simulink model "gm_parallel_lht"  (R2019b)
settings: Solver=FixedStepDiscrete  StartTime=0.0  StopTime=inf  RelTol=1e-3
undefined symbols (not defined in the file or in its folder): bt, height, width
libraries: hdlsllib x190, simulink x13, hdlmdlgenlib x7, dspsrcs4 x1
(part 17 of 18)

== system gm_parallel_lht/Parallel LHT/Parallel LHT Kernel/Hough Kernel/Hough Kernel Symmetric Look Ahead/Look Ahead Hough/Register Bank_instance42 ==
  Data In : Inport  OutDataTypeStr=fixdt(1, 11, 0)  PortDimensions=1  SampleTime=6.66666666666667e-09
  Write Enable : Inport  Port=2  OutDataTypeStr=boolean  PortDimensions=1  SampleTime=6.66666666666667e-09
  Delay_Switch : Switch  Criteria=u2 ~= 0  Threshold=double(0)  OutDataTypeStr=fixdt(1, 11, 0)  SampleTime=6.66666666666667e-09
  Unit Delay Enabled Synchronous_lowered : Delay  DelayLength=double(1)  InitialCondition=0  SampleTime=6.66666666666667e-09
  Data Out : Outport
  wires:
  Delay_Switch/1 -> Unit Delay Enabled Synchronous_lowered/1
  Write Enable/1 -> Delay_Switch/2
  Data In/1 -> Delay_Switch/1
  Unit Delay Enabled Synchronous_lowered/1 -> Delay_Switch/3, Data Out/1

== system gm_parallel_lht/Parallel LHT/Parallel LHT Kernel/Hough Kernel/Hough Kernel Symmetric Look Ahead/Look Ahead Hough/Register Bank_instance43 ==
  Data In : Inport  OutDataTypeStr=fixdt(1, 11, 0)  PortDimensions=1  SampleTime=6.66666666666667e-09
  Write Enable : Inport  Port=2  OutDataTypeStr=boolean  PortDimensions=1  SampleTime=6.66666666666667e-09
  Delay_Switch : Switch  Criteria=u2 ~= 0  Threshold=double(0)  OutDataTypeStr=fixdt(1, 11, 0)  SampleTime=6.66666666666667e-09
  Unit Delay Enabled Synchronous_lowered : Delay  DelayLength=double(1)  InitialCondition=0  SampleTime=6.66666666666667e-09
  Data Out : Outport
  wires:
  Delay_Switch/1 -> Unit Delay Enabled Synchronous_lowered/1
  Write Enable/1 -> Delay_Switch/2
  Data In/1 -> Delay_Switch/1
  Unit Delay Enabled Synchronous_lowered/1 -> Delay_Switch/3, Data Out/1

== system gm_parallel_lht/Parallel LHT/Parallel LHT Kernel/Hough Kernel/Hough Kernel Symmetric Look Ahead/Look Ahead Hough/Register Bank_instance44 ==
  Data In : Inport  OutDataTypeStr=fixdt(1, 11, 0)  PortDimensions=1  SampleTime=6.66666666666667e-09
  Write Enable : Inport  Port=2  OutDataTypeStr=boolean  PortDimensions=1  SampleTime=6.66666666666667e-09
  Delay_Switch : Switch  Criteria=u2 ~= 0  Threshold=double(0)  OutDataTypeStr=fixdt(1, 11, 0)  SampleTime=6.66666666666667e-09
  Unit Delay Enabled Synchronous_lowered : Delay  DelayLength=double(1)  InitialCondition=0  SampleTime=6.66666666666667e-09
  Data Out : Outport
  wires:
  Delay_Switch/1 -> Unit Delay Enabled Synchronous_lowered/1
  Write Enable/1 -> Delay_Switch/2
  Data In/1 -> Delay_Switch/1
  Unit Delay Enabled Synchronous_lowered/1 -> Delay_Switch/3, Data Out/1

== system gm_parallel_lht/Parallel LHT/Parallel LHT Kernel/Hough Kernel/Hough Kernel Symmetric Look Ahead/Look Ahead Hough/Register Bank_instance45 ==
  Data In : Inport  OutDataTypeStr=fixdt(1, 11, 0)  PortDimensions=1  SampleTime=6.66666666666667e-09
  Write Enable : Inport  Port=2  OutDataTypeStr=boolean  PortDimensions=1  SampleTime=6.66666666666667e-09
  Delay_Switch : Switch  Criteria=u2 ~= 0  Threshold=double(0)  OutDataTypeStr=fixdt(1, 11, 0)  SampleTime=6.66666666666667e-09
  Unit Delay Enabled Synchronous_lowered : Delay  DelayLength=double(1)  InitialCondition=0  SampleTime=6.66666666666667e-09
  Data Out : Outport
  wires:
  Delay_Switch/1 -> Unit Delay Enabled Synchronous_lowered/1
  Write Enable/1 -> Delay_Switch/2
  Data In/1 -> Delay_Switch/1
  Unit Delay Enabled Synchronous_lowered/1 -> Delay_Switch/3, Data Out/1

== system gm_parallel_lht/Parallel LHT/Parallel LHT Kernel/Hough Kernel/Hough Kernel Symmetric Look Ahead/Look Ahead Hough/Register Bank_instance46 ==
  Data In : Inport  OutDataTypeStr=fixdt(1, 11, 0)  PortDimensions=1  SampleTime=6.66666666666667e-09
  Write Enable : Inport  Port=2  OutDataTypeStr=boolean  PortDimensions=1  SampleTime=6.66666666666667e-09
  Delay_Switch : Switch  Criteria=u2 ~= 0  Threshold=double(0)  OutDataTypeStr=fixdt(1, 11, 0)  SampleTime=6.66666666666667e-09
  Unit Delay Enabled Synchronous_lowered : Delay  DelayLength=double(1)  InitialCondition=0  SampleTime=6.66666666666667e-09
  Data Out : Outport
  wires:
  Delay_Switch/1 -> Unit Delay Enabled Synchronous_lowered/1
  Write Enable/1 -> Delay_Switch/2
  Data In/1 -> Delay_Switch/1
  Unit Delay Enabled Synchronous_lowered/1 -> Delay_Switch/3, Data Out/1

== system gm_parallel_lht/Parallel LHT/Parallel LHT Kernel/Hough Kernel/Hough Kernel Symmetric Look Ahead/Look Ahead Hough/Register Bank_instance47 ==
  Data In : Inport  OutDataTypeStr=fixdt(1, 11, 0)  PortDimensions=1  SampleTime=6.66666666666667e-09
  Write Enable : Inport  Port=2  OutDataTypeStr=boolean  PortDimensions=1  SampleTime=6.66666666666667e-09
  Delay_Switch : Switch  Criteria=u2 ~= 0  Threshold=double(0)  OutDataTypeStr=fixdt(1, 11, 0)  SampleTime=6.66666666666667e-09
  Unit Delay Enabled Synchronous_lowered : Delay  DelayLength=double(1)  InitialCondition=0  SampleTime=6.66666666666667e-09
  Data Out : Outport
  wires:
  Delay_Switch/1 -> Unit Delay Enabled Synchronous_lowered/1
  Write Enable/1 -> Delay_Switch/2
  Data In/1 -> Delay_Switch/1
  Unit Delay Enabled Synchronous_lowered/1 -> Delay_Switch/3, Data Out/1

== system gm_parallel_lht/Parallel LHT/Parallel LHT Kernel/Hough Kernel/Hough Kernel Symmetric Look Ahead/Look Ahead Hough/Register Bank_instance48 ==
  Data In : Inport  OutDataTypeStr=fixdt(1, 11, 0)  PortDimensions=1  SampleTime=6.66666666666667e-09
  Write Enable : Inport  Port=2  OutDataTypeStr=boolean  PortDimensions=1  SampleTime=6.66666666666667e-09
  Delay_Switch : Switch  Criteria=u2 ~= 0  Threshold=double(0)  OutDataTypeStr=fixdt(1, 11, 0)  SampleTime=6.66666666666667e-09
  Unit Delay Enabled Synchronous_lowered : Delay  DelayLength=double(1)  InitialCondition=0  SampleTime=6.66666666666667e-09
  Data Out : Outport
  wires:
  Delay_Switch/1 -> Unit Delay Enabled Synchronous_lowered/1
  Write Enable/1 -> Delay_Switch/2
  Data In/1 -> Delay_Switch/1
  Unit Delay Enabled Synchronous_lowered/1 -> Delay_Switch/3, Data Out/1

== system gm_parallel_lht/Parallel LHT/Parallel LHT Kernel/Hough Kernel/Hough Kernel Symmetric Look Ahead/Look Ahead Hough/Register Bank_instance49 ==
  Data In : Inport  OutDataTypeStr=fixdt(1, 11, 0)  PortDimensions=1  SampleTime=6.66666666666667e-09
  Write Enable : Inport  Port=2  OutDataTypeStr=boolean  PortDimensions=1  SampleTime=6.66666666666667e-09
  Delay_Switch : Switch  Criteria=u2 ~= 0  Threshold=double(0)  OutDataTypeStr=fixdt(1, 11, 0)  SampleTime=6.66666666666667e-09
  Unit Delay Enabled Synchronous_lowered : Delay  DelayLength=double(1)  InitialCondition=0  SampleTime=6.66666666666667e-09
  Data Out : Outport
  wires:
  Delay_Switch/1 -> Unit Delay Enabled Synchronous_lowered/1
  Write Enable/1 -> Delay_Switch/2
  Data In/1 -> Delay_Switch/1
  Unit Delay Enabled Synchronous_lowered/1 -> Delay_Switch/3, Data Out/1

== system gm_parallel_lht/Parallel LHT/Parallel LHT Kernel/Hough Kernel/Hough Kernel Symmetric Look Ahead/Look Ahead Hough/Register Bank_instance5 ==
  Data In : Inport  OutDataTypeStr=fixdt(1, 11, 0)  PortDimensions=1  SampleTime=6.66666666666667e-09
  Write Enable : Inport  Port=2  OutDataTypeStr=boolean  PortDimensions=1  SampleTime=6.66666666666667e-09
  Delay_Switch : Switch  Criteria=u2 ~= 0  Threshold=double(0)  OutDataTypeStr=fixdt(1, 11, 0)  SampleTime=6.66666666666667e-09
  Unit Delay Enabled Synchronous_lowered : Delay  DelayLength=double(1)  InitialCondition=0  SampleTime=6.66666666666667e-09
  Data Out : Outport
  wires:
  Delay_Switch/1 -> Unit Delay Enabled Synchronous_lowered/1
  Write Enable/1 -> Delay_Switch/2
  Data In/1 -> Delay_Switch/1
  Unit Delay Enabled Synchronous_lowered/1 -> Delay_Switch/3, Data Out/1

== system gm_parallel_lht/Parallel LHT/Parallel LHT Kernel/Hough Kernel/Hough Kernel Symmetric Look Ahead/Look Ahead Hough/Register Bank_instance50 ==
  Data In : Inport  OutDataTypeStr=fixdt(1, 11, 0)  PortDimensions=1  SampleTime=6.66666666666667e-09
  Write Enable : Inport  Port=2  OutDataTypeStr=boolean  PortDimensions=1  SampleTime=6.66666666666667e-09
  Delay_Switch : Switch  Criteria=u2 ~= 0  Threshold=double(0)  OutDataTypeStr=fixdt(1, 11, 0)  SampleTime=6.66666666666667e-09
  Unit Delay Enabled Synchronous_lowered : Delay  DelayLength=double(1)  InitialCondition=0  SampleTime=6.66666666666667e-09
  Data Out : Outport
  wires:
  Delay_Switch/1 -> Unit Delay Enabled Synchronous_lowered/1
  Write Enable/1 -> Delay_Switch/2
  Data In/1 -> Delay_Switch/1
  Unit Delay Enabled Synchronous_lowered/1 -> Delay_Switch/3, Data Out/1

== system gm_parallel_lht/Parallel LHT/Parallel LHT Kernel/Hough Kernel/Hough Kernel Symmetric Look Ahead/Look Ahead Hough/Register Bank_instance51 ==
  Data In : Inport  OutDataTypeStr=fixdt(1, 11, 0)  PortDimensions=1  SampleTime=6.66666666666667e-09
  Write Enable : Inport  Port=2  OutDataTypeStr=boolean  PortDimensions=1  SampleTime=6.66666666666667e-09
  Delay_Switch : Switch  Criteria=u2 ~= 0  Threshold=double(0)  OutDataTypeStr=fixdt(1, 11, 0)  SampleTime=6.66666666666667e-09
  Unit Delay Enabled Synchronous_lowered : Delay  DelayLength=double(1)  InitialCondition=0  SampleTime=6.66666666666667e-09
  Data Out : Outport
  wires:
  Delay_Switch/1 -> Unit Delay Enabled Synchronous_lowered/1
  Write Enable/1 -> Delay_Switch/2
  Data In/1 -> Delay_Switch/1
  Unit Delay Enabled Synchronous_lowered/1 -> Delay_Switch/3, Data Out/1

== system gm_parallel_lht/Parallel LHT/Parallel LHT Kernel/Hough Kernel/Hough Kernel Symmetric Look Ahead/Look Ahead Hough/Register Bank_instance52 ==
  Data In : Inport  OutDataTypeStr=fixdt(1, 11, 0)  PortDimensions=1  SampleTime=6.66666666666667e-09
  Write Enable : Inport  Port=2  OutDataTypeStr=boolean  PortDimensions=1  SampleTime=6.66666666666667e-09
  Delay_Switch : Switch  Criteria=u2 ~= 0  Threshold=double(0)  OutDataTypeStr=fixdt(1, 11, 0)  SampleTime=6.66666666666667e-09
  Unit Delay Enabled Synchronous_lowered : Delay  DelayLength=double(1)  InitialCondition=0  SampleTime=6.66666666666667e-09
  Data Out : Outport
  wires:
  Delay_Switch/1 -> Unit Delay Enabled Synchronous_lowered/1
  Write Enable/1 -> Delay_Switch/2
  Data In/1 -> Delay_Switch/1
  Unit Delay Enabled Synchronous_lowered/1 -> Delay_Switch/3, Data Out/1

== system gm_parallel_lht/Parallel LHT/Parallel LHT Kernel/Hough Kernel/Hough Kernel Symmetric Look Ahead/Look Ahead Hough/Register Bank_instance53 ==
  Data In : Inport  OutDataTypeStr=fixdt(1, 11, 0)  PortDimensions=1  SampleTime=6.66666666666667e-09
  Write Enable : Inport  Port=2  OutDataTypeStr=boolean  PortDimensions=1  SampleTime=6.66666666666667e-09
  Delay_Switch : Switch  Criteria=u2 ~= 0  Threshold=double(0)  OutDataTypeStr=fixdt(1, 11, 0)  SampleTime=6.66666666666667e-09
  Unit Delay Enabled Synchronous_lowered : Delay  DelayLength=double(1)  InitialCondition=0  SampleTime=6.66666666666667e-09
  Data Out : Outport
  wires:
  Delay_Switch/1 -> Unit Delay Enabled Synchronous_lowered/1
  Write Enable/1 -> Delay_Switch/2
  Data In/1 -> Delay_Switch/1
  Unit Delay Enabled Synchronous_lowered/1 -> Delay_Switch/3, Data Out/1

== system gm_parallel_lht/Parallel LHT/Parallel LHT Kernel/Hough Kernel/Hough Kernel Symmetric Look Ahead/Look Ahead Hough/Register Bank_instance54 ==
  Data In : Inport  OutDataTypeStr=fixdt(1, 11, 0)  PortDimensions=1  SampleTime=6.66666666666667e-09
  Write Enable : Inport  Port=2  OutDataTypeStr=boolean  PortDimensions=1  SampleTime=6.66666666666667e-09
  Delay_Switch : Switch  Criteria=u2 ~= 0  Threshold=double(0)  OutDataTypeStr=fixdt(1, 11, 0)  SampleTime=6.66666666666667e-09
  Unit Delay Enabled Synchronous_lowered : Delay  DelayLength=double(1)  InitialCondition=0  SampleTime=6.66666666666667e-09
  Data Out : Outport
  wires:
  Delay_Switch/1 -> Unit Delay Enabled Synchronous_lowered/1
  Write Enable/1 -> Delay_Switch/2
  Data In/1 -> Delay_Switch/1
  Unit Delay Enabled Synchronous_lowered/1 -> Delay_Switch/3, Data Out/1

== system gm_parallel_lht/Parallel LHT/Parallel LHT Kernel/Hough Kernel/Hough Kernel Symmetric Look Ahead/Look Ahead Hough/Register Bank_instance55 ==
  Data In : Inport  OutDataTypeStr=fixdt(1, 11, 0)  PortDimensions=1  SampleTime=6.66666666666667e-09
  Write Enable : Inport  Port=2  OutDataTypeStr=boolean  PortDimensions=1  SampleTime=6.66666666666667e-09
  Delay_Switch : Switch  Criteria=u2 ~= 0  Threshold=double(0)  OutDataTypeStr=fixdt(1, 11, 0)  SampleTime=6.66666666666667e-09
  Unit Delay Enabled Synchronous_lowered : Delay  DelayLength=double(1)  InitialCondition=0  SampleTime=6.66666666666667e-09
  Data Out : Outport
  wires:
  Delay_Switch/1 -> Unit Delay Enabled Synchronous_lowered/1
  Write Enable/1 -> Delay_Switch/2
  Data In/1 -> Delay_Switch/1
  Unit Delay Enabled Synchronous_lowered/1 -> Delay_Switch/3, Data Out/1

== system gm_parallel_lht/Parallel LHT/Parallel LHT Kernel/Hough Kernel/Hough Kernel Symmetric Look Ahead/Look Ahead Hough/Register Bank_instance56 ==
  Data In : Inport  OutDataTypeStr=fixdt(1, 11, 0)  PortDimensions=1  SampleTime=6.66666666666667e-09
  Write Enable : Inport  Port=2  OutDataTypeStr=boolean  PortDimensions=1  SampleTime=6.66666666666667e-09
  Delay_Switch : Switch  Criteria=u2 ~= 0  Threshold=double(0)  OutDataTypeStr=fixdt(1, 11, 0)  SampleTime=6.66666666666667e-09
  Unit Delay Enabled Synchronous_lowered : Delay  DelayLength=double(1)  InitialCondition=0  SampleTime=6.66666666666667e-09
  Data Out : Outport
  wires:
  Delay_Switch/1 -> Unit Delay Enabled Synchronous_lowered/1
  Write Enable/1 -> Delay_Switch/2
  Data In/1 -> Delay_Switch/1
  Unit Delay Enabled Synchronous_lowered/1 -> Delay_Switch/3, Data Out/1

== system gm_parallel_lht/Parallel LHT/Parallel LHT Kernel/Hough Kernel/Hough Kernel Symmetric Look Ahead/Look Ahead Hough/Register Bank_instance57 ==
  Data In : Inport  OutDataTypeStr=fixdt(1, 11, 0)  PortDimensions=1  SampleTime=6.66666666666667e-09
  Write Enable : Inport  Port=2  OutDataTypeStr=boolean  PortDimensions=1  SampleTime=6.66666666666667e-09
  Delay_Switch : Switch  Criteria=u2 ~= 0  Threshold=double(0)  OutDataTypeStr=fixdt(1, 11, 0)  SampleTime=6.66666666666667e-09
  Unit Delay Enabled Synchronous_lowered : Delay  DelayLength=double(1)  InitialCondition=0  SampleTime=6.66666666666667e-09
  Data Out : Outport
  wires:
  Delay_Switch/1 -> Unit Delay Enabled Synchronous_lowered/1
  Write Enable/1 -> Delay_Switch/2
  Data In/1 -> Delay_Switch/1
  Unit Delay Enabled Synchronous_lowered/1 -> Delay_Switch/3, Data Out/1

== system gm_parallel_lht/Parallel LHT/Parallel LHT Kernel/Hough Kernel/Hough Kernel Symmetric Look Ahead/Look Ahead Hough/Register Bank_instance58 ==
  Data In : Inport  OutDataTypeStr=fixdt(1, 11, 0)  PortDimensions=1  SampleTime=6.66666666666667e-09
  Write Enable : Inport  Port=2  OutDataTypeStr=boolean  PortDimensions=1  SampleTime=6.66666666666667e-09
  Delay_Switch : Switch  Criteria=u2 ~= 0  Threshold=double(0)  OutDataTypeStr=fixdt(1, 11, 0)  SampleTime=6.66666666666667e-09
  Unit Delay Enabled Synchronous_lowered : Delay  DelayLength=double(1)  InitialCondition=0  SampleTime=6.66666666666667e-09
  Data Out : Outport
  wires:
  Delay_Switch/1 -> Unit Delay Enabled Synchronous_lowered/1
  Write Enable/1 -> Delay_Switch/2
  Data In/1 -> Delay_Switch/1
  Unit Delay Enabled Synchronous_lowered/1 -> Delay_Switch/3, Data Out/1

== system gm_parallel_lht/Parallel LHT/Parallel LHT Kernel/Hough Kernel/Hough Kernel Symmetric Look Ahead/Look Ahead Hough/Register Bank_instance59 ==
  Data In : Inport  OutDataTypeStr=fixdt(1, 11, 0)  PortDimensions=1  SampleTime=6.66666666666667e-09
  Write Enable : Inport  Port=2  OutDataTypeStr=boolean  PortDimensions=1  SampleTime=6.66666666666667e-09
  Delay_Switch : Switch  Criteria=u2 ~= 0  Threshold=double(0)  OutDataTypeStr=fixdt(1, 11, 0)  SampleTime=6.66666666666667e-09
  Unit Delay Enabled Synchronous_lowered : Delay  DelayLength=double(1)  InitialCondition=0  SampleTime=6.66666666666667e-09
  Data Out : Outport
  wires:
  Delay_Switch/1 -> Unit Delay Enabled Synchronous_lowered/1
  Write Enable/1 -> Delay_Switch/2
  Data In/1 -> Delay_Switch/1
  Unit Delay Enabled Synchronous_lowered/1 -> Delay_Switch/3, Data Out/1

== system gm_parallel_lht/Parallel LHT/Parallel LHT Kernel/Hough Kernel/Hough Kernel Symmetric Look Ahead/Look Ahead Hough/Register Bank_instance6 ==
  Data In : Inport  OutDataTypeStr=fixdt(1, 11, 0)  PortDimensions=1  SampleTime=6.66666666666667e-09
  Write Enable : Inport  Port=2  OutDataTypeStr=boolean  PortDimensions=1  SampleTime=6.66666666666667e-09
  Delay_Switch : Switch  Criteria=u2 ~= 0  Threshold=double(0)  OutDataTypeStr=fixdt(1, 11, 0)  SampleTime=6.66666666666667e-09
  Unit Delay Enabled Synchronous_lowered : Delay  DelayLength=double(1)  InitialCondition=0  SampleTime=6.66666666666667e-09
  Data Out : Outport
  wires:
  Delay_Switch/1 -> Unit Delay Enabled Synchronous_lowered/1
  Write Enable/1 -> Delay_Switch/2
  Data In/1 -> Delay_Switch/1
  Unit Delay Enabled Synchronous_lowered/1 -> Delay_Switch/3, Data Out/1

== system gm_parallel_lht/Parallel LHT/Parallel LHT Kernel/Hough Kernel/Hough Kernel Symmetric Look Ahead/Look Ahead Hough/Register Bank_instance60 ==
  Data In : Inport  OutDataTypeStr=fixdt(1, 11, 0)  PortDimensions=1  SampleTime=6.66666666666667e-09
  Write Enable : Inport  Port=2  OutDataTypeStr=boolean  PortDimensions=1  SampleTime=6.66666666666667e-09
  Delay_Switch : Switch  Criteria=u2 ~= 0  Threshold=double(0)  OutDataTypeStr=fixdt(1, 11, 0)  SampleTime=6.66666666666667e-09
  Unit Delay Enabled Synchronous_lowered : Delay  DelayLength=double(1)  InitialCondition=0  SampleTime=6.66666666666667e-09
  Data Out : Outport
  wires:
  Delay_Switch/1 -> Unit Delay Enabled Synchronous_lowered/1
  Write Enable/1 -> Delay_Switch/2
  Data In/1 -> Delay_Switch/1
  Unit Delay Enabled Synchronous_lowered/1 -> Delay_Switch/3, Data Out/1

== system gm_parallel_lht/Parallel LHT/Parallel LHT Kernel/Hough Kernel/Hough Kernel Symmetric Look Ahead/Look Ahead Hough/Register Bank_instance61 ==
  Data In : Inport  OutDataTypeStr=fixdt(1, 11, 0)  PortDimensions=1  SampleTime=6.66666666666667e-09
  Write Enable : Inport  Port=2  OutDataTypeStr=boolean  PortDimensions=1  SampleTime=6.66666666666667e-09
  Delay_Switch : Switch  Criteria=u2 ~= 0  Threshold=double(0)  OutDataTypeStr=fixdt(1, 11, 0)  SampleTime=6.66666666666667e-09
  Unit Delay Enabled Synchronous_lowered : Delay  DelayLength=double(1)  InitialCondition=0  SampleTime=6.66666666666667e-09
  Data Out : Outport
  wires:
  Delay_Switch/1 -> Unit Delay Enabled Synchronous_lowered/1
  Write Enable/1 -> Delay_Switch/2
  Data In/1 -> Delay_Switch/1
  Unit Delay Enabled Synchronous_lowered/1 -> Delay_Switch/3, Data Out/1

== system gm_parallel_lht/Parallel LHT/Parallel LHT Kernel/Hough Kernel/Hough Kernel Symmetric Look Ahead/Look Ahead Hough/Register Bank_instance62 ==
  Data In : Inport  OutDataTypeStr=fixdt(1, 11, 0)  PortDimensions=1  SampleTime=6.66666666666667e-09
  Write Enable : Inport  Port=2  OutDataTypeStr=boolean  PortDimensions=1  SampleTime=6.66666666666667e-09
  Delay_Switch : Switch  Criteria=u2 ~= 0  Threshold=double(0)  OutDataTypeStr=fixdt(1, 11, 0)  SampleTime=6.66666666666667e-09
  Unit Delay Enabled Synchronous_lowered : Delay  DelayLength=double(1)  InitialCondition=0  SampleTime=6.66666666666667e-09
  Data Out : Outport
  wires:
  Delay_Switch/1 -> Unit Delay Enabled Synchronous_lowered/1
  Write Enable/1 -> Delay_Switch/2
  Data In/1 -> Delay_Switch/1
  Unit Delay Enabled Synchronous_lowered/1 -> Delay_Switch/3, Data Out/1

== system gm_parallel_lht/Parallel LHT/Parallel LHT Kernel/Hough Kernel/Hough Kernel Symmetric Look Ahead/Look Ahead Hough/Register Bank_instance63 ==
  Data In : Inport  OutDataTypeStr=fixdt(1, 11, 0)  PortDimensions=1  SampleTime=6.66666666666667e-09
  Write Enable : Inport  Port=2  OutDataTypeStr=boolean  PortDimensions=1  SampleTime=6.66666666666667e-09
  Delay_Switch : Switch  Criteria=u2 ~= 0  Threshold=double(0)  OutDataTypeStr=fixdt(1, 11, 0)  SampleTime=6.66666666666667e-09
  Unit Delay Enabled Synchronous_lowered : Delay  DelayLength=double(1)  InitialCondition=0  SampleTime=6.66666666666667e-09
  Data Out : Outport
  wires:
  Delay_Switch/1 -> Unit Delay Enabled Synchronous_lowered/1
  Write Enable/1 -> Delay_Switch/2
  Data In/1 -> Delay_Switch/1
  Unit Delay Enabled Synchronous_lowered/1 -> Delay_Switch/3, Data Out/1

== system gm_parallel_lht/Parallel LHT/Parallel LHT Kernel/Hough Kernel/Hough Kernel Symmetric Look Ahead/Look Ahead Hough/Register Bank_instance64 ==
  Data In : Inport  OutDataTypeStr=fixdt(1, 11, 0)  PortDimensions=1  SampleTime=6.66666666666667e-09
  Write Enable : Inport  Port=2  OutDataTypeStr=boolean  PortDimensions=1  SampleTime=6.66666666666667e-09
  Delay_Switch : Switch  Criteria=u2 ~= 0  Threshold=double(0)  OutDataTypeStr=fixdt(1, 11, 0)  SampleTime=6.66666666666667e-09
  Unit Delay Enabled Synchronous_lowered : Delay  DelayLength=double(1)  InitialCondition=0  SampleTime=6.66666666666667e-09
  Data Out : Outport
  wires:
  Delay_Switch/1 -> Unit Delay Enabled Synchronous_lowered/1
  Write Enable/1 -> Delay_Switch/2
  Data In/1 -> Delay_Switch/1
  Unit Delay Enabled Synchronous_lowered/1 -> Delay_Switch/3, Data Out/1

== system gm_parallel_lht/Parallel LHT/Parallel LHT Kernel/Hough Kernel/Hough Kernel Symmetric Look Ahead/Look Ahead Hough/Register Bank_instance65 ==
  Data In : Inport  OutDataTypeStr=fixdt(1, 11, 0)  PortDimensions=1  SampleTime=6.66666666666667e-09
  Write Enable : Inport  Port=2  OutDataTypeStr=boolean  PortDimensions=1  SampleTime=6.66666666666667e-09
  Delay_Switch : Switch  Criteria=u2 ~= 0  Threshold=double(0)  OutDataTypeStr=fixdt(1, 11, 0)  SampleTime=6.66666666666667e-09
  Unit Delay Enabled Synchronous_lowered : Delay  DelayLength=double(1)  InitialCondition=0  SampleTime=6.66666666666667e-09
  Data Out : Outport
  wires:
  Delay_Switch/1 -> Unit Delay Enabled Synchronous_lowered/1
  Write Enable/1 -> Delay_Switch/2
  Data In/1 -> Delay_Switch/1
  Unit Delay Enabled Synchronous_lowered/1 -> Delay_Switch/3, Data Out/1

== system gm_parallel_lht/Parallel LHT/Parallel LHT Kernel/Hough Kernel/Hough Kernel Symmetric Look Ahead/Look Ahead Hough/Register Bank_instance66 ==
  Data In : Inport  OutDataTypeStr=fixdt(1, 11, 0)  PortDimensions=1  SampleTime=6.66666666666667e-09
  Write Enable : Inport  Port=2  OutDataTypeStr=boolean  PortDimensions=1  SampleTime=6.66666666666667e-09
  Delay_Switch : Switch  Criteria=u2 ~= 0  Threshold=double(0)  OutDataTypeStr=fixdt(1, 11, 0)  SampleTime=6.66666666666667e-09
  Unit Delay Enabled Synchronous_lowered : Delay  DelayLength=double(1)  InitialCondition=0  SampleTime=6.66666666666667e-09
  Data Out : Outport
  wires:
  Delay_Switch/1 -> Unit Delay Enabled Synchronous_lowered/1
  Write Enable/1 -> Delay_Switch/2
  Data In/1 -> Delay_Switch/1
  Unit Delay Enabled Synchronous_lowered/1 -> Delay_Switch/3, Data Out/1

== system gm_parallel_lht/Parallel LHT/Parallel LHT Kernel/Hough Kernel/Hough Kernel Symmetric Look Ahead/Look Ahead Hough/Register Bank_instance67 ==
  Data In : Inport  OutDataTypeStr=fixdt(1, 11, 0)  PortDimensions=1  SampleTime=6.66666666666667e-09
  Write Enable : Inport  Port=2  OutDataTypeStr=boolean  PortDimensions=1  SampleTime=6.66666666666667e-09
  Delay_Switch : Switch  Criteria=u2 ~= 0  Threshold=double(0)  OutDataTypeStr=fixdt(1, 11, 0)  SampleTime=6.66666666666667e-09
  Unit Delay Enabled Synchronous_lowered : Delay  DelayLength=double(1)  InitialCondition=0  SampleTime=6.66666666666667e-09
  Data Out : Outport
  wires:
  Delay_Switch/1 -> Unit Delay Enabled Synchronous_lowered/1
  Write Enable/1 -> Delay_Switch/2
  Data In/1 -> Delay_Switch/1
  Unit Delay Enabled Synchronous_lowered/1 -> Delay_Switch/3, Data Out/1

== system gm_parallel_lht/Parallel LHT/Parallel LHT Kernel/Hough Kernel/Hough Kernel Symmetric Look Ahead/Look Ahead Hough/Register Bank_instance68 ==
  Data In : Inport  OutDataTypeStr=fixdt(1, 11, 0)  PortDimensions=1  SampleTime=6.66666666666667e-09
  Write Enable : Inport  Port=2  OutDataTypeStr=boolean  PortDimensions=1  SampleTime=6.66666666666667e-09
  Delay_Switch : Switch  Criteria=u2 ~= 0  Threshold=double(0)  OutDataTypeStr=fixdt(1, 11, 0)  SampleTime=6.66666666666667e-09
  Unit Delay Enabled Synchronous_lowered : Delay  DelayLength=double(1)  InitialCondition=0  SampleTime=6.66666666666667e-09
  Data Out : Outport
  wires:
  Delay_Switch/1 -> Unit Delay Enabled Synchronous_lowered/1
  Write Enable/1 -> Delay_Switch/2
  Data In/1 -> Delay_Switch/1
  Unit Delay Enabled Synchronous_lowered/1 -> Delay_Switch/3, Data Out/1

== system gm_parallel_lht/Parallel LHT/Parallel LHT Kernel/Hough Kernel/Hough Kernel Symmetric Look Ahead/Look Ahead Hough/Register Bank_instance69 ==
  Data In : Inport  OutDataTypeStr=fixdt(1, 11, 0)  PortDimensions=1  SampleTime=6.66666666666667e-09
  Write Enable : Inport  Port=2  OutDataTypeStr=boolean  PortDimensions=1  SampleTime=6.66666666666667e-09
  Delay_Switch : Switch  Criteria=u2 ~= 0  Threshold=double(0)  OutDataTypeStr=fixdt(1, 11, 0)  SampleTime=6.66666666666667e-09
  Unit Delay Enabled Synchronous_lowered : Delay  DelayLength=double(1)  InitialCondition=0  SampleTime=6.66666666666667e-09
  Data Out : Outport
  wires:
  Delay_Switch/1 -> Unit Delay Enabled Synchronous_lowered/1
  Write Enable/1 -> Delay_Switch/2
  Data In/1 -> Delay_Switch/1
  Unit Delay Enabled Synchronous_lowered/1 -> Delay_Switch/3, Data Out/1

== system gm_parallel_lht/Parallel LHT/Parallel LHT Kernel/Hough Kernel/Hough Kernel Symmetric Look Ahead/Look Ahead Hough/Register Bank_instance7 ==
  Data In : Inport  OutDataTypeStr=fixdt(1, 11, 0)  PortDimensions=1  SampleTime=6.66666666666667e-09
  Write Enable : Inport  Port=2  OutDataTypeStr=boolean  PortDimensions=1  SampleTime=6.66666666666667e-09
  Delay_Switch : Switch  Criteria=u2 ~= 0  Threshold=double(0)  OutDataTypeStr=fixdt(1, 11, 0)  SampleTime=6.66666666666667e-09
  Unit Delay Enabled Synchronous_lowered : Delay  DelayLength=double(1)  InitialCondition=0  SampleTime=6.66666666666667e-09
  Data Out : Outport
  wires:
  Delay_Switch/1 -> Unit Delay Enabled Synchronous_lowered/1
  Write Enable/1 -> Delay_Switch/2
  Data In/1 -> Delay_Switch/1
  Unit Delay Enabled Synchronous_lowered/1 -> Delay_Switch/3, Data Out/1

== system gm_parallel_lht/Parallel LHT/Parallel LHT Kernel/Hough Kernel/Hough Kernel Symmetric Look Ahead/Look Ahead Hough/Register Bank_instance70 ==
  Data In : Inport  OutDataTypeStr=fixdt(1, 11, 0)  PortDimensions=1  SampleTime=6.66666666666667e-09
  Write Enable : Inport  Port=2  OutDataTypeStr=boolean  PortDimensions=1  SampleTime=6.66666666666667e-09
  Delay_Switch : Switch  Criteria=u2 ~= 0  Threshold=double(0)  OutDataTypeStr=fixdt(1, 11, 0)  SampleTime=6.66666666666667e-09
  Unit Delay Enabled Synchronous_lowered : Delay  DelayLength=double(1)  InitialCondition=0  SampleTime=6.66666666666667e-09
  Data Out : Outport
  wires:
  Delay_Switch/1 -> Unit Delay Enabled Synchronous_lowered/1
  Write Enable/1 -> Delay_Switch/2
  Data In/1 -> Delay_Switch/1
  Unit Delay Enabled Synchronous_lowered/1 -> Delay_Switch/3, Data Out/1

== system gm_parallel_lht/Parallel LHT/Parallel LHT Kernel/Hough Kernel/Hough Kernel Symmetric Look Ahead/Look Ahead Hough/Register Bank_instance71 ==
  Data In : Inport  OutDataTypeStr=fixdt(1, 11, 0)  PortDimensions=1  SampleTime=6.66666666666667e-09
  Write Enable : Inport  Port=2  OutDataTypeStr=boolean  PortDimensions=1  SampleTime=6.66666666666667e-09
  Delay_Switch : Switch  Criteria=u2 ~= 0  Threshold=double(0)  OutDataTypeStr=fixdt(1, 11, 0)  SampleTime=6.66666666666667e-09
  Unit Delay Enabled Synchronous_lowered : Delay  DelayLength=double(1)  InitialCondition=0  SampleTime=6.66666666666667e-09
  Data Out : Outport
  wires:
  Delay_Switch/1 -> Unit Delay Enabled Synchronous_lowered/1
  Write Enable/1 -> Delay_Switch/2
  Data In/1 -> Delay_Switch/1
  Unit Delay Enabled Synchronous_lowered/1 -> Delay_Switch/3, Data Out/1

== system gm_parallel_lht/Parallel LHT/Parallel LHT Kernel/Hough Kernel/Hough Kernel Symmetric Look Ahead/Look Ahead Hough/Register Bank_instance72 ==
  Data In : Inport  OutDataTypeStr=fixdt(1, 11, 0)  PortDimensions=1  SampleTime=6.66666666666667e-09
  Write Enable : Inport  Port=2  OutDataTypeStr=boolean  PortDimensions=1  SampleTime=6.66666666666667e-09
  Delay_Switch : Switch  Criteria=u2 ~= 0  Threshold=double(0)  OutDataTypeStr=fixdt(1, 11, 0)  SampleTime=6.66666666666667e-09
  Unit Delay Enabled Synchronous_lowered : Delay  DelayLength=double(1)  InitialCondition=0  SampleTime=6.66666666666667e-09
  Data Out : Outport
  wires:
  Delay_Switch/1 -> Unit Delay Enabled Synchronous_lowered/1
  Write Enable/1 -> Delay_Switch/2
  Data In/1 -> Delay_Switch/1
  Unit Delay Enabled Synchronous_lowered/1 -> Delay_Switch/3, Data Out/1

== system gm_parallel_lht/Parallel LHT/Parallel LHT Kernel/Hough Kernel/Hough Kernel Symmetric Look Ahead/Look Ahead Hough/Register Bank_instance73 ==
  Data In : Inport  OutDataTypeStr=fixdt(1, 11, 0)  PortDimensions=1  SampleTime=6.66666666666667e-09
  Write Enable : Inport  Port=2  OutDataTypeStr=boolean  PortDimensions=1  SampleTime=6.66666666666667e-09
  Delay_Switch : Switch  Criteria=u2 ~= 0  Threshold=double(0)  OutDataTypeStr=fixdt(1, 11, 0)  SampleTime=6.66666666666667e-09
  Unit Delay Enabled Synchronous_lowered : Delay  DelayLength=double(1)  InitialCondition=0  SampleTime=6.66666666666667e-09
  Data Out : Outport
  wires:
  Delay_Switch/1 -> Unit Delay Enabled Synchronous_lowered/1
  Write Enable/1 -> Delay_Switch/2
  Data In/1 -> Delay_Switch/1
  Unit Delay Enabled Synchronous_lowered/1 -> Delay_Switch/3, Data Out/1

== system gm_parallel_lht/Parallel LHT/Parallel LHT Kernel/Hough Kernel/Hough Kernel Symmetric Look Ahead/Look Ahead Hough/Register Bank_instance74 ==
  Data In : Inport  OutDataTypeStr=fixdt(1, 11, 0)  PortDimensions=1  SampleTime=6.66666666666667e-09
  Write Enable : Inport  Port=2  OutDataTypeStr=boolean  PortDimensions=1  SampleTime=6.66666666666667e-09
  Delay_Switch : Switch  Criteria=u2 ~= 0  Threshold=double(0)  OutDataTypeStr=fixdt(1, 11, 0)  SampleTime=6.66666666666667e-09
  Unit Delay Enabled Synchronous_lowered : Delay  DelayLength=double(1)  InitialCondition=0  SampleTime=6.66666666666667e-09
  Data Out : Outport
  wires:
  Delay_Switch/1 -> Unit Delay Enabled Synchronous_lowered/1
  Write Enable/1 -> Delay_Switch/2
  Data In/1 -> Delay_Switch/1
  Unit Delay Enabled Synchronous_lowered/1 -> Delay_Switch/3, Data Out/1

== system gm_parallel_lht/Parallel LHT/Parallel LHT Kernel/Hough Kernel/Hough Kernel Symmetric Look Ahead/Look Ahead Hough/Register Bank_instance75 ==
  Data In : Inport  OutDataTypeStr=fixdt(1, 11, 0)  PortDimensions=1  SampleTime=6.66666666666667e-09
  Write Enable : Inport  Port=2  OutDataTypeStr=boolean  PortDimensions=1  SampleTime=6.66666666666667e-09
  Delay_Switch : Switch  Criteria=u2 ~= 0  Threshold=double(0)  OutDataTypeStr=fixdt(1, 11, 0)  SampleTime=6.66666666666667e-09
  Unit Delay Enabled Synchronous_lowered : Delay  DelayLength=double(1)  InitialCondition=0  SampleTime=6.66666666666667e-09
  Data Out : Outport
  wires:
  Delay_Switch/1 -> Unit Delay Enabled Synchronous_lowered/1
  Write Enable/1 -> Delay_Switch/2
  Data In/1 -> Delay_Switch/1
  Unit Delay Enabled Synchronous_lowered/1 -> Delay_Switch/3, Data Out/1

== system gm_parallel_lht/Parallel LHT/Parallel LHT Kernel/Hough Kernel/Hough Kernel Symmetric Look Ahead/Look Ahead Hough/Register Bank_instance76 ==
  Data In : Inport  OutDataTypeStr=fixdt(1, 11, 0)  PortDimensions=1  SampleTime=6.66666666666667e-09
  Write Enable : Inport  Port=2  OutDataTypeStr=boolean  PortDimensions=1  SampleTime=6.66666666666667e-09
  Delay_Switch : Switch  Criteria=u2 ~= 0  Threshold=double(0)  OutDataTypeStr=fixdt(1, 11, 0)  SampleTime=6.66666666666667e-09
  Unit Delay Enabled Synchronous_lowered : Delay  DelayLength=double(1)  InitialCondition=0  SampleTime=6.66666666666667e-09
  Data Out : Outport
  wires:
  Delay_Switch/1 -> Unit Delay Enabled Synchronous_lowered/1
  Write Enable/1 -> Delay_Switch/2
  Data In/1 -> Delay_Switch/1
  Unit Delay Enabled Synchronous_lowered/1 -> Delay_Switch/3, Data Out/1

== system gm_parallel_lht/Parallel LHT/Parallel LHT Kernel/Hough Kernel/Hough Kernel Symmetric Look Ahead/Look Ahead Hough/Register Bank_instance77 ==
  Data In : Inport  OutDataTypeStr=fixdt(1, 11, 0)  PortDimensions=1  SampleTime=6.66666666666667e-09
  Write Enable : Inport  Port=2  OutDataTypeStr=boolean  PortDimensions=1  SampleTime=6.66666666666667e-09
  Delay_Switch : Switch  Criteria=u2 ~= 0  Threshold=double(0)  OutDataTypeStr=fixdt(1, 11, 0)  SampleTime=6.66666666666667e-09
  Unit Delay Enabled Synchronous_lowered : Delay  DelayLength=double(1)  InitialCondition=0  SampleTime=6.66666666666667e-09
  Data Out : Outport
  wires:
  Delay_Switch/1 -> Unit Delay Enabled Synchronous_lowered/1
  Write Enable/1 -> Delay_Switch/2
  Data In/1 -> Delay_Switch/1
  Unit Delay Enabled Synchronous_lowered/1 -> Delay_Switch/3, Data Out/1

== system gm_parallel_lht/Parallel LHT/Parallel LHT Kernel/Hough Kernel/Hough Kernel Symmetric Look Ahead/Look Ahead Hough/Register Bank_instance78 ==
  Data In : Inport  OutDataTypeStr=fixdt(1, 11, 0)  PortDimensions=1  SampleTime=6.66666666666667e-09
  Write Enable : Inport  Port=2  OutDataTypeStr=boolean  PortDimensions=1  SampleTime=6.66666666666667e-09
  Delay_Switch : Switch  Criteria=u2 ~= 0  Threshold=double(0)  OutDataTypeStr=fixdt(1, 11, 0)  SampleTime=6.66666666666667e-09
  Unit Delay Enabled Synchronous_lowered : Delay  DelayLength=double(1)  InitialCondition=0  SampleTime=6.66666666666667e-09
  Data Out : Outport
  wires:
  Delay_Switch/1 -> Unit Delay Enabled Synchronous_lowered/1
  Write Enable/1 -> Delay_Switch/2
  Data In/1 -> Delay_Switch/1
  Unit Delay Enabled Synchronous_lowered/1 -> Delay_Switch/3, Data Out/1

== system gm_parallel_lht/Parallel LHT/Parallel LHT Kernel/Hough Kernel/Hough Kernel Symmetric Look Ahead/Look Ahead Hough/Register Bank_instance79 ==
  Data In : Inport  OutDataTypeStr=fixdt(1, 11, 0)  PortDimensions=1  SampleTime=6.66666666666667e-09
  Write Enable : Inport  Port=2  OutDataTypeStr=boolean  PortDimensions=1  SampleTime=6.66666666666667e-09
  Delay_Switch : Switch  Criteria=u2 ~= 0  Threshold=double(0)  OutDataTypeStr=fixdt(1, 11, 0)  SampleTime=6.66666666666667e-09
  Unit Delay Enabled Synchronous_lowered : Delay  DelayLength=double(1)  InitialCondition=0  SampleTime=6.66666666666667e-09
  Data Out : Outport
  wires:
  Delay_Switch/1 -> Unit Delay Enabled Synchronous_lowered/1
  Write Enable/1 -> Delay_Switch/2
  Data In/1 -> Delay_Switch/1
  Unit Delay Enabled Synchronous_lowered/1 -> Delay_Switch/3, Data Out/1

== system gm_parallel_lht/Parallel LHT/Parallel LHT Kernel/Hough Kernel/Hough Kernel Symmetric Look Ahead/Look Ahead Hough/Register Bank_instance8 ==
  Data In : Inport  OutDataTypeStr=fixdt(1, 11, 0)  PortDimensions=1  SampleTime=6.66666666666667e-09
  Write Enable : Inport  Port=2  OutDataTypeStr=boolean  PortDimensions=1  SampleTime=6.66666666666667e-09
  Delay_Switch : Switch  Criteria=u2 ~= 0  Threshold=double(0)  OutDataTypeStr=fixdt(1, 11, 0)  SampleTime=6.66666666666667e-09
  Unit Delay Enabled Synchronous_lowered : Delay  DelayLength=double(1)  InitialCondition=0  SampleTime=6.66666666666667e-09
  Data Out : Outport
  wires:
  Delay_Switch/1 -> Unit Delay Enabled Synchronous_lowered/1
  Write Enable/1 -> Delay_Switch/2
  Data In/1 -> Delay_Switch/1
  Unit Delay Enabled Synchronous_lowered/1 -> Delay_Switch/3, Data Out/1

== system gm_parallel_lht/Parallel LHT/Parallel LHT Kernel/Hough Kernel/Hough Kernel Symmetric Look Ahead/Look Ahead Hough/Register Bank_instance80 ==
  Data In : Inport  OutDataTypeStr=fixdt(1, 11, 0)  PortDimensions=1  SampleTime=6.66666666666667e-09
  Write Enable : Inport  Port=2  OutDataTypeStr=boolean  PortDimensions=1  SampleTime=6.66666666666667e-09
  Delay_Switch : Switch  Criteria=u2 ~= 0  Threshold=double(0)  OutDataTypeStr=fixdt(1, 11, 0)  SampleTime=6.66666666666667e-09
  Unit Delay Enabled Synchronous_lowered : Delay  DelayLength=double(1)  InitialCondition=0  SampleTime=6.66666666666667e-09
  Data Out : Outport
  wires:
  Delay_Switch/1 -> Unit Delay Enabled Synchronous_lowered/1
  Write Enable/1 -> Delay_Switch/2
  Data In/1 -> Delay_Switch/1
  Unit Delay Enabled Synchronous_lowered/1 -> Delay_Switch/3, Data Out/1

== system gm_parallel_lht/Parallel LHT/Parallel LHT Kernel/Hough Kernel/Hough Kernel Symmetric Look Ahead/Look Ahead Hough/Register Bank_instance81 ==
  Data In : Inport  OutDataTypeStr=fixdt(1, 11, 0)  PortDimensions=1  SampleTime=6.66666666666667e-09
  Write Enable : Inport  Port=2  OutDataTypeStr=boolean  PortDimensions=1  SampleTime=6.66666666666667e-09
  Delay_Switch : Switch  Criteria=u2 ~= 0  Threshold=double(0)  OutDataTypeStr=fixdt(1, 11, 0)  SampleTime=6.66666666666667e-09
  Unit Delay Enabled Synchronous_lowered : Delay  DelayLength=double(1)  InitialCondition=0  SampleTime=6.66666666666667e-09
  Data Out : Outport
  wires:
  Delay_Switch/1 -> Unit Delay Enabled Synchronous_lowered/1
  Write Enable/1 -> Delay_Switch/2
  Data In/1 -> Delay_Switch/1
  Unit Delay Enabled Synchronous_lowered/1 -> Delay_Switch/3, Data Out/1

== system gm_parallel_lht/Parallel LHT/Parallel LHT Kernel/Hough Kernel/Hough Kernel Symmetric Look Ahead/Look Ahead Hough/Register Bank_instance82 ==
  Data In : Inport  OutDataTypeStr=fixdt(1, 11, 0)  PortDimensions=1  SampleTime=6.66666666666667e-09
  Write Enable : Inport  Port=2  OutDataTypeStr=boolean  PortDimensions=1  SampleTime=6.66666666666667e-09
  Delay_Switch : Switch  Criteria=u2 ~= 0  Threshold=double(0)  OutDataTypeStr=fixdt(1, 11, 0)  SampleTime=6.66666666666667e-09
  Unit Delay Enabled Synchronous_lowered : Delay  DelayLength=double(1)  InitialCondition=0  SampleTime=6.66666666666667e-09
  Data Out : Outport
  wires:
  Delay_Switch/1 -> Unit Delay Enabled Synchronous_lowered/1
  Write Enable/1 -> Delay_Switch/2
  Data In/1 -> Delay_Switch/1
  Unit Delay Enabled Synchronous_lowered/1 -> Delay_Switch/3, Data Out/1

== system gm_parallel_lht/Parallel LHT/Parallel LHT Kernel/Hough Kernel/Hough Kernel Symmetric Look Ahead/Look Ahead Hough/Register Bank_instance83 ==
  Data In : Inport  OutDataTypeStr=fixdt(1, 11, 0)  PortDimensions=1  SampleTime=6.66666666666667e-09
  Write Enable : Inport  Port=2  OutDataTypeStr=boolean  PortDimensions=1  SampleTime=6.66666666666667e-09
  Delay_Switch : Switch  Criteria=u2 ~= 0  Threshold=double(0)  OutDataTypeStr=fixdt(1, 11, 0)  SampleTime=6.66666666666667e-09
  Unit Delay Enabled Synchronous_lowered : Delay  DelayLength=double(1)  InitialCondition=0  SampleTime=6.66666666666667e-09
  Data Out : Outport
  wires:
  Delay_Switch/1 -> Unit Delay Enabled Synchronous_lowered/1
  Write Enable/1 -> Delay_Switch/2
  Data In/1 -> Delay_Switch/1
  Unit Delay Enabled Synchronous_lowered/1 -> Delay_Switch/3, Data Out/1

== system gm_parallel_lht/Parallel LHT/Parallel LHT Kernel/Hough Kernel/Hough Kernel Symmetric Look Ahead/Look Ahead Hough/Register Bank_instance84 ==
  Data In : Inport  OutDataTypeStr=fixdt(1, 11, 0)  PortDimensions=1  SampleTime=6.66666666666667e-09
  Write Enable : Inport  Port=2  OutDataTypeStr=boolean  PortDimensions=1  SampleTime=6.66666666666667e-09
  Delay_Switch : Switch  Criteria=u2 ~= 0  Threshold=double(0)  OutDataTypeStr=fixdt(1, 11, 0)  SampleTime=6.66666666666667e-09
  Unit Delay Enabled Synchronous_lowered : Delay  DelayLength=double(1)  InitialCondition=0  SampleTime=6.66666666666667e-09
  Data Out : Outport
  wires:
  Delay_Switch/1 -> Unit Delay Enabled Synchronous_lowered/1
  Write Enable/1 -> Delay_Switch/2
  Data In/1 -> Delay_Switch/1
  Unit Delay Enabled Synchronous_lowered/1 -> Delay_Switch/3, Data Out/1

== system gm_parallel_lht/Parallel LHT/Parallel LHT Kernel/Hough Kernel/Hough Kernel Symmetric Look Ahead/Look Ahead Hough/Register Bank_instance85 ==
  Data In : Inport  OutDataTypeStr=fixdt(1, 11, 0)  PortDimensions=1  SampleTime=6.66666666666667e-09
  Write Enable : Inport  Port=2  OutDataTypeStr=boolean  PortDimensions=1  SampleTime=6.66666666666667e-09
  Delay_Switch : Switch  Criteria=u2 ~= 0  Threshold=double(0)  OutDataTypeStr=fixdt(1, 11, 0)  SampleTime=6.66666666666667e-09
  Unit Delay Enabled Synchronous_lowered : Delay  DelayLength=double(1)  InitialCondition=0  SampleTime=6.66666666666667e-09
  Data Out : Outport
  wires:
  Delay_Switch/1 -> Unit Delay Enabled Synchronous_lowered/1
  Write Enable/1 -> Delay_Switch/2
  Data In/1 -> Delay_Switch/1
  Unit Delay Enabled Synchronous_lowered/1 -> Delay_Switch/3, Data Out/1

== system gm_parallel_lht/Parallel LHT/Parallel LHT Kernel/Hough Kernel/Hough Kernel Symmetric Look Ahead/Look Ahead Hough/Register Bank_instance86 ==
  Data In : Inport  OutDataTypeStr=fixdt(1, 11, 0)  PortDimensions=1  SampleTime=6.66666666666667e-09
  Write Enable : Inport  Port=2  OutDataTypeStr=boolean  PortDimensions=1  SampleTime=6.66666666666667e-09
  Delay_Switch : Switch  Criteria=u2 ~= 0  Threshold=double(0)  OutDataTypeStr=fixdt(1, 11, 0)  SampleTime=6.66666666666667e-09
  Unit Delay Enabled Synchronous_lowered : Delay  DelayLength=double(1)  InitialCondition=0  SampleTime=6.66666666666667e-09
  Data Out : Outport
  wires:
  Delay_Switch/1 -> Unit Delay Enabled Synchronous_lowered/1
  Write Enable/1 -> Delay_Switch/2
  Data In/1 -> Delay_Switch/1
  Unit Delay Enabled Synchronous_lowered/1 -> Delay_Switch/3, Data Out/1

== system gm_parallel_lht/Parallel LHT/Parallel LHT Kernel/Hough Kernel/Hough Kernel Symmetric Look Ahead/Look Ahead Hough/Register Bank_instance87 ==
  Data In : Inport  OutDataTypeStr=fixdt(1, 11, 0)  PortDimensions=1  SampleTime=6.66666666666667e-09
  Write Enable : Inport  Port=2  OutDataTypeStr=boolean  PortDimensions=1  SampleTime=6.66666666666667e-09
  Delay_Switch : Switch  Criteria=u2 ~= 0  Threshold=double(0)  OutDataTypeStr=fixdt(1, 11, 0)  SampleTime=6.66666666666667e-09
  Unit Delay Enabled Synchronous_lowered : Delay  DelayLength=double(1)  InitialCondition=0  SampleTime=6.66666666666667e-09
  Data Out : Outport
  wires:
  Delay_Switch/1 -> Unit Delay Enabled Synchronous_lowered/1
  Write Enable/1 -> Delay_Switch/2
  Data In/1 -> Delay_Switch/1
  Unit Delay Enabled Synchronous_lowered/1 -> Delay_Switch/3, Data Out/1

== system gm_parallel_lht/Parallel LHT/Parallel LHT Kernel/Hough Kernel/Hough Kernel Symmetric Look Ahead/Look Ahead Hough/Register Bank_instance88 ==
  Data In : Inport  OutDataTypeStr=fixdt(1, 11, 0)  PortDimensions=1  SampleTime=6.66666666666667e-09
  Write Enable : Inport  Port=2  OutDataTypeStr=boolean  PortDimensions=1  SampleTime=6.66666666666667e-09
  Delay_Switch : Switch  Criteria=u2 ~= 0  Threshold=double(0)  OutDataTypeStr=fixdt(1, 11, 0)  SampleTime=6.66666666666667e-09
  Unit Delay Enabled Synchronous_lowered : Delay  DelayLength=double(1)  InitialCondition=0  SampleTime=6.66666666666667e-09
  Data Out : Outport
  wires:
  Delay_Switch/1 -> Unit Delay Enabled Synchronous_lowered/1
  Write Enable/1 -> Delay_Switch/2
  Data In/1 -> Delay_Switch/1
  Unit Delay Enabled Synchronous_lowered/1 -> Delay_Switch/3, Data Out/1

== system gm_parallel_lht/Parallel LHT/Parallel LHT Kernel/Hough Kernel/Hough Kernel Symmetric Look Ahead/Look Ahead Hough/Register Bank_instance89 ==
  Data In : Inport  OutDataTypeStr=fixdt(1, 11, 0)  PortDimensions=1  SampleTime=6.66666666666667e-09
  Write Enable : Inport  Port=2  OutDataTypeStr=boolean  PortDimensions=1  SampleTime=6.66666666666667e-09
  Delay_Switch : Switch  Criteria=u2 ~= 0  Threshold=double(0)  OutDataTypeStr=fixdt(1, 11, 0)  SampleTime=6.66666666666667e-09
  Unit Delay Enabled Synchronous_lowered : Delay  DelayLength=double(1)  InitialCondition=0  SampleTime=6.66666666666667e-09
  Data Out : Outport
  wires:
  Delay_Switch/1 -> Unit Delay Enabled Synchronous_lowered/1
  Write Enable/1 -> Delay_Switch/2
  Data In/1 -> Delay_Switch/1
  Unit Delay Enabled Synchronous_lowered/1 -> Delay_Switch/3, Data Out/1

== system gm_parallel_lht/Parallel LHT/Parallel LHT Kernel/Hough Kernel/Hough Kernel Symmetric Look Ahead/Look Ahead Hough/Register Bank_instance9 ==
  Data In : Inport  OutDataTypeStr=fixdt(1, 11, 0)  PortDimensions=1  SampleTime=6.66666666666667e-09
  Write Enable : Inport  Port=2  OutDataTypeStr=boolean  PortDimensions=1  SampleTime=6.66666666666667e-09
  Delay_Switch : Switch  Criteria=u2 ~= 0  Threshold=double(0)  OutDataTypeStr=fixdt(1, 11, 0)  SampleTime=6.66666666666667e-09
  Unit Delay Enabled Synchronous_lowered : Delay  DelayLength=double(1)  InitialCondition=0  SampleTime=6.66666666666667e-09
  Data Out : Outport
  wires:
  Delay_Switch/1 -> Unit Delay Enabled Synchronous_lowered/1
  Write Enable/1 -> Delay_Switch/2
  Data In/1 -> Delay_Switch/1
  Unit Delay Enabled Synchronous_lowered/1 -> Delay_Switch/3, Data Out/1

== system gm_parallel_lht/Parallel LHT/Parallel LHT Kernel/Hough Kernel/Hough Kernel Symmetric Look Ahead/Look Ahead Hough/Register Bank_instance90 ==
  Data In : Inport  OutDataTypeStr=fixdt(1, 11, 0)  PortDimensions=1  SampleTime=6.66666666666667e-09
  Write Enable : Inport  Port=2  OutDataTypeStr=boolean  PortDimensions=1  SampleTime=6.66666666666667e-09
  Delay_Switch : Switch  Criteria=u2 ~= 0  Threshold=double(0)  OutDataTypeStr=fixdt(1, 11, 0)  SampleTime=6.66666666666667e-09
  Unit Delay Enabled Synchronous_lowered : Delay  DelayLength=double(1)  InitialCondition=0  SampleTime=6.66666666666667e-09
  Data Out : Outport
  wires:
  Delay_Switch/1 -> Unit Delay Enabled Synchronous_lowered/1
  Write Enable/1 -> Delay_Switch/2
  Data In/1 -> Delay_Switch/1
  Unit Delay Enabled Synchronous_lowered/1 -> Delay_Switch/3, Data Out/1

== system gm_parallel_lht/Parallel LHT/Parallel LHT Kernel/Hough Kernel/Hough Kernel Symmetric Look Ahead/Look Ahead Hough/Register Bank_instance91 ==
  Data In : Inport  OutDataTypeStr=fixdt(1, 11, 0)  PortDimensions=1  SampleTime=6.66666666666667e-09
  Write Enable : Inport  Port=2  OutDataTypeStr=boolean  PortDimensions=1  SampleTime=6.66666666666667e-09
  Delay_Switch : Switch  Criteria=u2 ~= 0  Threshold=double(0)  OutDataTypeStr=fixdt(1, 11, 0)  SampleTime=6.66666666666667e-09
  Unit Delay Enabled Synchronous_lowered : Delay  DelayLength=double(1)  InitialCondition=0  SampleTime=6.66666666666667e-09
  Data Out : Outport
  wires:
  Delay_Switch/1 -> Unit Delay Enabled Synchronous_lowered/1
  Write Enable/1 -> Delay_Switch/2
  Data In/1 -> Delay_Switch/1
  Unit Delay Enabled Synchronous_lowered/1 -> Delay_Switch/3, Data Out/1

== matlab function gm_parallel_lht/Parallel LHT/Parallel LHT Accumulator/Accumulator Controller/Accumulator Controller ==
  data: sof input; mode output; eof input; read output; clear output; index output; ntheta input; nrho input; valid output
function [mode, read, clear, index, valid] = fcn(sof, eof, ntheta, nrho)

IDLE = fi(0, 0, 2, 0);
VOTE = fi(1, 0, 2, 0);
READ = fi(2, 0, 2, 0);
CLEAR = fi(3, 0, 2, 0);

persistent current_state;
persistent rho_counter;
persistent theta_counter;

if isempty(current_state)
    current_state = IDLE;
end

if isempty(rho_counter)
    rho_counter = fi(0, 0, 16, 0);
end

if isempty(theta_counter)
    theta_counter = fi(0, 0, 16, 0);
end

switch current_state
    case IDLE
        rho_counter = fi(0, 0, 16, 0);
        theta_counter = fi(0, 0, 16, 0);
        
        clear = false;
        read = rho_counter;
        index = theta_counter;
        valid = false;
        
        if sof
            mode = true;
            current_state = VOTE;
        else
            mode = false;
            current_state = IDLE;
        end
        
    case VOTE
        rho_counter = fi(0, 0, 16, 0);
        theta_counter = fi(0, 0, 16, 0);
        
        mode = true;
        clear = false;
        valid = false;
        
        read = rho_counter;
        index = theta_counter;
        
        if eof
            current_state = READ;
        else
            current_state = VOTE;
        end
        
    case READ
        mode = false;
        clear = false;
        read = rho_counter;
        index = theta_counter;
        valid = true;
        
        if theta_counter >= nrho && rho_counter >= ntheta
            rho_counter = fi(0, 0, 16, 0);
            theta_counter = fi(0, 0, 16, 0);
            current_state = CLEAR;
        elseif rho_counter >= nrho
            theta_counter = fi(theta_counter + 1, 0, 16, 0);
            rho_counter = fi(0, 0, 16, 0);
            current_state = READ;
        else
            rho_counter = fi(rho_counter + 1, 0, 16, 0);
            current_state = READ;
        end
        
    case CLEAR
        mode = false;
        clear = true;
        valid = false;
        
        read = rho_counter;
        index = theta_counter;
        
        if rho_counter >= nrho
            rho_counter = fi(0, 0, 16, 0);
            theta_counter = fi(0, 0, 16, 0);
            current_state = IDLE;
        else
            rho_counter = fi(rho_counter + 1, 0, 16, 0);
            theta_counter = fi(0, 0, 16, 0);
            current_state = CLEAR;
        end
        
    otherwise
        rho_counter = fi(0, 0, 16, 0);
        theta_counter = fi(0, 0, 16, 0);
        
        mode = false;
        clear = false;
        valid = false;
        
        read = rho_counter;
        index = theta_counter;
        
        current_state = IDLE;
        
end
